simulink subsystem "ADC"  (R2024b)
settings: Solver=VariableStepAuto  StartTime=0.0  StopTime=10.0  RelTol=1e-3
values from neighbouring files (symbols this model uses):
  Ts = 0.001    [Plant_ModelParameters.m]
undefined symbols (not defined in the file or in its folder): daq
settings Model: Creator=Riccardo Grosso  LastModifiedBy=Federico Bergami

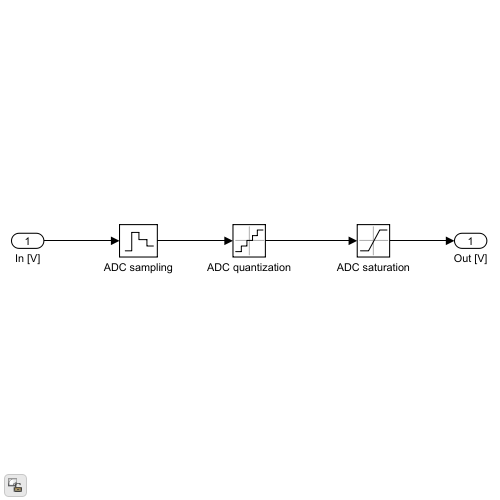
[thumbnail: Simulink's stored preview of the top-level diagram]
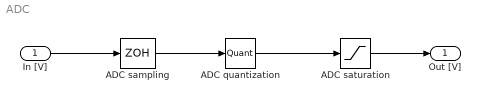
== system ADC ==
  In [V] : Inport
  ADC quantization : Quantizer  QuantizationInterval=daq.adc.q
  ADC sampling : ZeroOrderHold  SampleTime=Ts
  ADC saturation : Saturate  UpperLimit=daq.adc.fs  LowerLimit=-daq.adc.fs  ZeroCross=off
  Out [V] : Outport  Unit=V
  wires:
  ADC quantization/1 -> ADC saturation/1
  ADC sampling/1 -> ADC quantization/1
  In [V]/1 -> ADC sampling/1
  ADC saturation/1 -> Out [V]/1
